simulink model "k1visbs"  (Simulink 8.5)
settings: Solver=ode45  StartTime=0.0  StopTime=10.0  RelTol=1e-3
libraries: cdsAdcx0 x1, TYPEC_MASTER x1, cdsEpicsOut x1, dac x1, cdsIPCx x1, cdsParameters x1
settings Model: Creator=controls  LastModifiedBy=controls
settings DataIOCC: SignalLoggingSaveFormat=Dataset
settings OptimizationCC: ExpressionDepthLimit=128
settings DebuggingCC: UnderspecifiedInitializationDetection=Simplified  MergeDetectMultiDrivingBlocksExec=error  FcnCallInpInsideContextMsg=EnableAllAsError  StateNameClashWarn=none
settings GRTTargetCC: CombineOutputUpdateFcns=on  GRTInterface=off

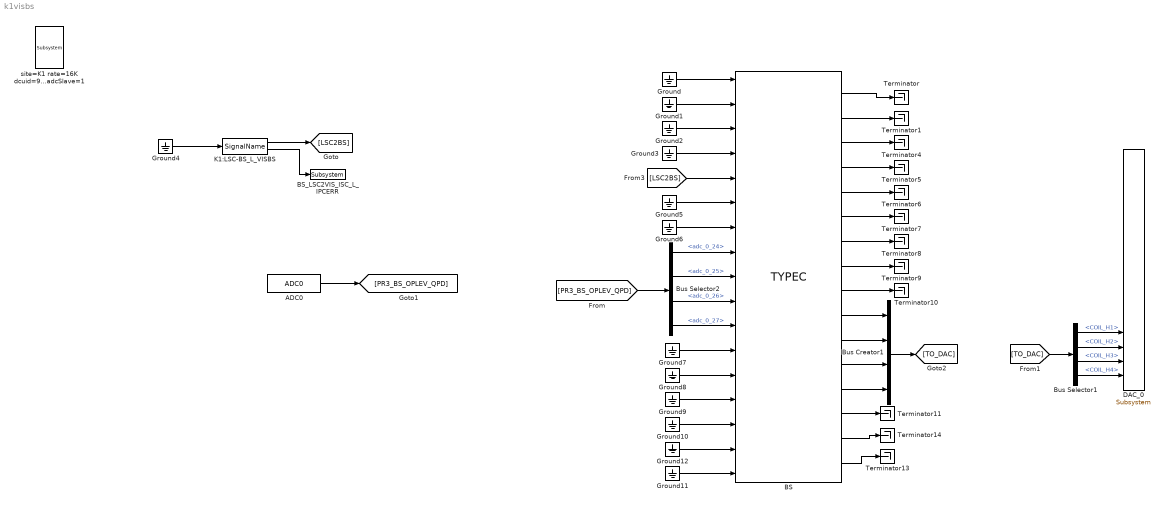
== system k1visbs ==
  ADC0 : cdsAdcx0/ADC0  Tag=cdsAdc  Description=|
      | type-GSC_16AI64SSA
      | card_num=0
      settings: AttributesFormatString=%<Description>\n%<Tag>
  BS : TYPEC_MASTER/TYPEC  Description=TYPEC MASTER
      settings: AttributesFormatString=%<Description>
  BS_LSC2VIS_ISC_L_IPCERR : cdsEpicsOut/Subsystem  Tag=cdsEpicsOutput  Description=|
      | Purpose:                                          
      | Output a FE signal to an EPICS channel.           
      |                                                   
      | Operation:                                        
      | Takes input value and passes it to EPICS record.  
      |                                                   
      | Usage:                                            
      | Name the part with the desired EPICS rrecord name.
      settings: AttributesFormatString=%<Tag>
  Bus Creator1 : BusCreator  Inputs='COIL_H1','COIL_H2','COIL_H3','COIL_H4'
  Bus Selector1 : BusSelector  Description=ADC Selector  OutputSignals=COIL_H1,COIL_H2,COIL_H3,COIL_H4
      settings: AttributesFormatString=%<Description>
  Bus Selector2 : BusSelector  Description=ADC Selector  OutputSignals=adc_0_24,adc_0_25,adc_0_26,adc_0_27
      settings: AttributesFormatString=%<Description>
  DAC_0 : dac/Subsystem  Description=|
      | type=GSC_16AO16,
      | card_num=0
      settings: AttributesFormatString=%<Description>
  Ground{,1..12} (13 alike) : Ground
  K1:LSC-BS_L_VISBS : cdsIPCx/SignalName  Tag=cdsIPCx_PCIE  Description=Inter-Process Communication via PCI Express network.
      settings: AttributesFormatString=%<Tag>
  Terminator{,1,4..11,13..14} (12 alike) : Terminator
  site=K1 rate=16K dcuid=96 host=k1pr2 specific_cpu=4 adcSlave=1 : cdsParameters/Subsystem  Tag=cdsParameters  Description=|
      | Purpose:                                                                                                                                                                                                                                
      | Provide system parameters to the FE code generator to properly configure the generated EPICS names, rep rate of the FE controller, and the Data Acquisition node ID for proper storage of data from this FE controller.                 
      |                                                                                                                                                                                                                                         
      | Useage:                                                                                                                                                                                                                                 
      | The part NAME field is used to identify the FE parameters. It must be of the form:                                                                                                                                                      
      | site=                                                                                                                                                                                                                                   
      | rate=                                                                                                                                                                                                                                   
      | dcuid=                                                                                                                                                                                                                                  
      |                                                                                                                                                                                                                                         
      | Where:                                                                                                                                                                                                                                  
      | site= argument may be H1, H2, L1, M1, G1, either as a single argument or multiple, for example site=H1,H2. These are the only names allowed. These will become the first two characters of all EPICS and signal names (for example G1:).
      |                                                                                                                                                                                                                                         
      | rate= may be 2K, 16K, 32K, or 64K                                                                                                                                                                                                       
      |                                                                                                                                                                                                                                         
      | dcuid= is site specific ie it must be unique at each site.
      settings: AttributesFormatString=%<Tag>
  wires:
  Ground2/1 -> BS/3
  Ground1/1 -> BS/2
  Ground/1 -> BS/1
  Ground3/1 -> BS/4
  Ground8/1 -> BS/13
  Ground7/1 -> BS/12
  Ground9/1 -> BS/14
  Ground10/1 -> BS/15
  Ground5/1 -> BS/6
  Ground12/1 -> BS/16
  Ground11/1 -> BS/17
  BS/1 -> Terminator/1
  BS/2 -> Terminator1/1
  BS/5 -> Terminator6/1
  BS/4 -> Terminator5/1
  BS/6 -> Terminator7/1
  BS/3 -> Terminator4/1
  BS/7 -> Terminator8/1
  BS/9 -> Terminator10/1
  BS/8 -> Terminator9/1
  BS/14 -> Terminator11/1
  BS/15 -> Terminator14/1
  BS/16 -> Terminator13/1
  Ground6/1 -> BS/7
  Ground4/1 -> K1:LSC-BS_L_VISBS/1
  K1:LSC-BS_L_VISBS/2 -> BS_LSC2VIS_ISC_L_IPCERR/1
  K1:LSC-BS_L_VISBS/1 -> [LSC2BS]
  [LSC2BS] -> BS/5
  [PR3_BS_OPLEV_QPD] -> Bus Selector2/1
  Bus Selector2/1 -> BS/8  "<adc_0_24>"
  Bus Selector2/4 -> BS/11  "<adc_0_27>"
  Bus Selector2/3 -> BS/10  "<adc_0_26>"
  Bus Selector2/2 -> BS/9  "<adc_0_25>"
  BS/12 -> Bus Creator1/3
  BS/11 -> Bus Creator1/2
  BS/13 -> Bus Creator1/4
  BS/10 -> Bus Creator1/1
  Bus Creator1/1 -> [TO_DAC]
  [TO_DAC] -> Bus Selector1/1
  Bus Selector1/4 -> DAC_0/16  "<COIL_H4>"
  Bus Selector1/3 -> DAC_0/15  "<COIL_H3>"
  Bus Selector1/2 -> DAC_0/14  "<COIL_H2>"
  Bus Selector1/1 -> DAC_0/13  "<COIL_H1>"
  ADC0/1 -> [PR3_BS_OPLEV_QPD]
